simulink model "HDLInterpolator"  (R2024a)
settings: Solver=VariableStepAuto  StartTime=0.0  StopTime=stopTime  RelTol=1e-3
undefined symbols (not defined in the file): CONST
libraries: dspsrcs4 x2, HDL_ieee_8021513 x2, whdlutilities x1
settings Model: Creator=cotti  LastModifiedBy=cotti

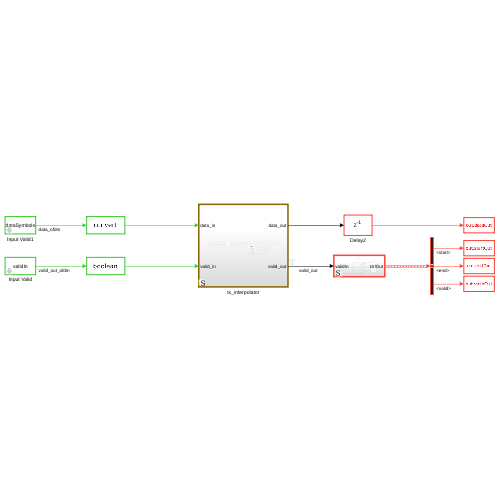
[thumbnail: Simulink's stored preview of the top-level diagram]
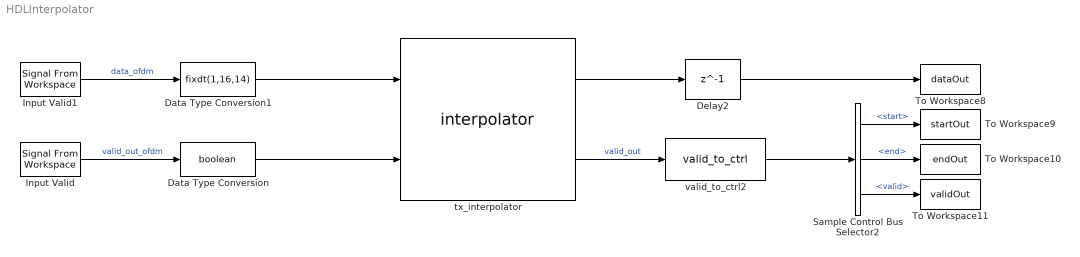
== system HDLInterpolator ==
  Data Type Conversion : DataTypeConversion  OutDataTypeStr=boolean  SaturateOnIntegerOverflow=off  RndMeth=Floor
  Data Type Conversion1 : DataTypeConversion  OutDataTypeStr=fixdt(1,16,14)  SaturateOnIntegerOverflow=off  RndMeth=Floor
  Delay2 : Delay  DelayLength=1  InitialCondition=0  UseCircularBuffer=on
  Input Valid : dspsrcs4/Signal From Workspace  X=validIn  Ts=1/CONST.fPHY  nsamps=1  OutputAfterFinalValue=Setting to zero  ignoreOrWarnInputAndFrameLengths=off  OutputFrames=off
  Input Valid1 : dspsrcs4/Signal From Workspace  X=dataSymbols  Ts=1/CONST.fPHY  nsamps=1  OutputAfterFinalValue=Setting to zero  ignoreOrWarnInputAndFrameLengths=off  OutputFrames=off
  Sample Control Bus Selector2 : whdlutilities/Sample Control Bus Selector  OutputSignals=start,end,valid
  To Workspace10 : ToWorkspace  VariableName=endOut  SampleTime=1/(CONST.fPHY*CONST.txL)
      settings: Save2DSignal=2-D array (concatenate along first dimension)
  To Workspace11 : ToWorkspace  VariableName=validOut  SampleTime=1/(CONST.fPHY*CONST.txL)
      settings: Save2DSignal=2-D array (concatenate along first dimension)
  To Workspace8 : ToWorkspace  VariableName=dataOut  SampleTime=1/(CONST.fPHY*CONST.txL)
      settings: Save2DSignal=2-D array (concatenate along first dimension)
  To Workspace9 : ToWorkspace  VariableName=startOut  SampleTime=1/(CONST.fPHY*CONST.txL)
      settings: Save2DSignal=2-D array (concatenate along first dimension)
  tx_interpolator : HDL_ieee_8021513/interpolator  SystemSampleTime=-1  VariantActivationTime=update diagram  AllowFlexibleInterface=on  Latency=0  AutoFrameSizeCalculation=off
      settings: SourceProductName=HDL IEEE 8021513
  valid_to_ctrl2 : HDL_ieee_8021513/valid_to_ctrl  SystemSampleTime=-1  VariantActivationTime=update diagram  AllowFlexibleInterface=on  Latency=0  AutoFrameSizeCalculation=off
      settings: SourceProductName=HDL IEEE 8021513
  wires:
  Delay2/1 -> To Workspace8/1
  Sample Control Bus Selector2/3 -> To Workspace11/1  "<valid>"
  Sample Control Bus Selector2/2 -> To Workspace10/1  "<end>"
  valid_to_ctrl2/1 -> Sample Control Bus Selector2/1
  Sample Control Bus Selector2/1 -> To Workspace9/1  "<start>"
  Input Valid/1 -> Data Type Conversion/1  "valid_out_ofdm"
  Input Valid1/1 -> Data Type Conversion1/1  "data_ofdm"
  Data Type Conversion/1 -> tx_interpolator/2
  Data Type Conversion1/1 -> tx_interpolator/1
  tx_interpolator/2 -> valid_to_ctrl2/1  "valid_out"
  tx_interpolator/1 -> Delay2/1
